simulink model "Batch_Model"  (R2023a)
settings: Solver=VariableStepAuto  StartTime=0.0  StopTime=10.0  RelTol=1e-3
libraries: NSA_DEVS_LOGISTICS_ATOMIC x2, NSA_DEVS_SINKS_ATOMIC x2, NSA_DEVS_SOURCES_ATOMIC x1
settings Model: Creator=david  LastModifiedBy=david

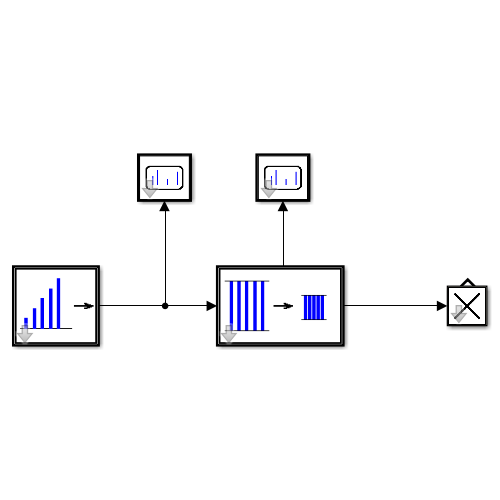
[thumbnail: Simulink's stored preview of the top-level diagram]
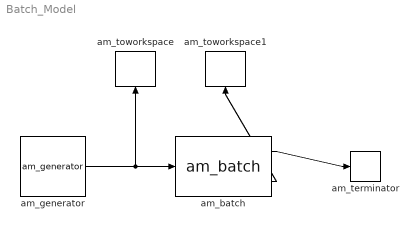
== system Batch_Model ==
  am_batch : NSA_DEVS_LOGISTICS_ATOMIC/am_batch  N=10  tau=[0,1]  debug=0
      settings: SourceProductName=NSA_DEVS
  am_generator : NSA_DEVS_SOURCES_ATOMIC/am_generator  tG=1  n0=1  nG=100  tau=[0,1]  debug=0
      settings: SourceProductName=NSA_DEVS
  am_terminator : NSA_DEVS_LOGISTICS_ATOMIC/am_terminator  tau=[0,1]  debug=0
      settings: SourceProductName=NSA_DEVS
  am_toworkspace : NSA_DEVS_SINKS_ATOMIC/am_toworkspace  varname="\"genOut\""  t0=0  format="\"vector\""  tau=[0,5]  debug=0
      settings: SourceProductName=NSA_DEVS
  am_toworkspace1 : NSA_DEVS_SINKS_ATOMIC/am_toworkspace  varname="\"batch_n\""  t0=0  format="\"vector\""  tau=[0,5]  debug=0
      settings: SourceProductName=NSA_DEVS
  wires:
  am_generator/1 -> am_toworkspace/1, am_batch/1
  am_batch/1 -> am_terminator/1
  am_batch/2 -> am_toworkspace1/1
